simulink model "rakete"  (R2017b)
settings: Solver=ode4  StartTime=0.0  StopTime=600.0  FixedStep=10  RelTol=1e-3
settings Model: Creator=squirrel  LastModifiedBy=squirrel

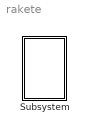
== system rakete ==
  Subsystem : Subsystem  mask{m1_leer=500, m2_leer=1000, St1_Treibstoff=4000, St2_Treibstoff=1500, Durchsatz_1=20, Durchsatz_2=15, SchubProDurchsatz=4000}

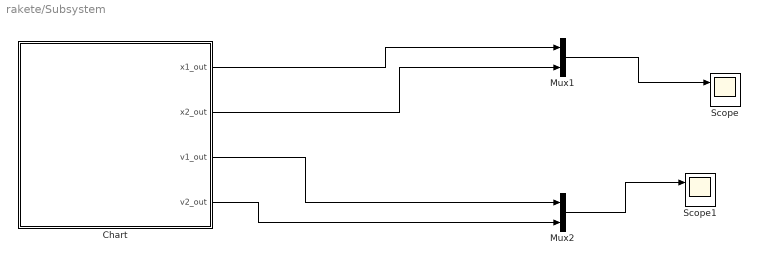
== system rakete/Subsystem ==
  Chart : Stateflow chart  TreatAsAtomicUnit=on
  Mux1 : Mux  Inputs=2
  Mux2 : Mux  Inputs=2
  Scope : Scope  NumInputPorts=2
  Scope1 : Scope  NumInputPorts=2
  wires:
  Mux1/1 -> Scope/1
  Chart/1(x1_out) -> Mux1/1
  Chart/2(x2_out) -> Mux1/2
  Chart/3(v1_out) -> Mux2/1
  Chart/4(v2_out) -> Mux2/2
  Mux2/1 -> Scope1/1

== stateflow chart rakete/Subsystem/Chart ==
  settings: updateMethod=CONTINUOUS
  state StufenGemeinsam
    du:
    %derivatives
    [v1_dot, v2_dot] = acc1();
    x1_dot = v1; x2_dot = v2;
    m1_dot = -Durchsatz_1; m2_dot = 0;
    %output
    x1_out = x1; x2_out = x2;
    v1_out = v1; v2_out = v2;
  state Stufe2Ausgebrannt
    du:
    %derivatives
    [v1_dot, v2_dot] = acc3();
    x1_dot = v1; x2_dot = v2;
    m1_dot = 0; m2_dot = 0;
    %output
    x1_out = x1; x2_out = x2;
    v1_out = v1; v2_out = v2;
  state StufenGetrennt
    du:
    %derivatives
    [v1_dot, v2_dot] = acc2();
    x1_dot = v1; x2_dot = v2;
    m1_dot = 0; m2_dot = -Durchsatz_2;
    %output
    x1_out = x1; x2_out = x2;
    v1_out = v1; v2_out = v2;
  (default) -> StufenGemeinsam : {init();}
  StufenGemeinsam -> StufenGetrennt : [m1 <= m1_leer]
  StufenGetrennt -> Stufe2Ausgebrannt : [m2 <= m2_leer]
  data: a1 function_output; a2 function_output; a1 function_output; a2 function_output; a1 function_output; a2 function_output; m1_leer parameter; m2_leer parameter; St1_Treibstoff parameter; St2_Treibstoff parameter; Durchsatz_1 parameter; Durchsatz_2 parameter; x2 local; v1 local; v2 local; m1 local; m2 local; x1_out output; x2_out output; v1_out output; v2_out output; SchubProDurchsatz parameter double; x1 local; er constant double =6378000; G constant double =66.743 * 10^(-12); me constant double =5.9736 * 10^24
  data x2 settings: updateMethod=SF_CONTINUOUS_TIME_DATA
  data v1 settings: updateMethod=SF_CONTINUOUS_TIME_DATA
  data v2 settings: updateMethod=SF_CONTINUOUS_TIME_DATA
  data m1 settings: updateMethod=SF_CONTINUOUS_TIME_DATA
  data m2 settings: updateMethod=SF_CONTINUOUS_TIME_DATA
  data x1 settings: updateMethod=SF_CONTINUOUS_TIME_DATA
  function init:
    | function init
    | v1 = 0; % Geschwindigkeit Stufe 1 [m/s]
    | v2 = 0; % Geschwindigkeit Stufe 2 [m/s]
    | 
    | m1 = m1_leer + St1_Treibstoff; % initiale Masse Stufe 1 [kg]
    | m2 = m2_leer + St2_Treibstoff; % initiale Masse Stufe 2 [kg]
    | x1 = 0; % Position Stufe 1
    | x2 = 0; % Position Stufe 2
  function [a1, a2] = acc1:
    | function [a1, a2] = acc1
    | 
    | m = m1 + m2 + m1_leer + m2_leer; % aktuelle Gesamtmasse Stufe 1 und 2 [kg]
    | Fg = (G * me * m) / ((er + x1)^2); % Potentialkraft [N]
    | Fs = Durchsatz_1 * SchubProDurchsatz; % Schubkraft [N]
    | 
    | a1 = (Fs - Fg) / m; % Beschleunigung Stufe 1 [m/s^2]
    | a2 = a1; % Beschleunigung Stufe 2 [m/s²]
  function [a1, a2] = acc2:
    | function [a1, a2] = acc2
    | 
    | m = m2 + m2_leer; % aktuelle Gesamtmasse Stufe 2 [kg]
    | 
    | Fg1 = (G * me) / (er + x1)^2; % Potentialkraft Stufe 1[N]
    | 
    | Fg2 = (G * me * m) / (er + x2)^2; % Potentialkraft Stufe 2[N]
    | Fs2 = Durchsatz_2 * SchubProDurchsatz;  % Schubkraft Stufe 2 [N]
    | a1 = - Fg1;  % Beschleunigung Stufe 1 [m/s²]
    | a2 = (Fs2 - Fg2) / m; % Beschleunigung Stufe 2 [m/s²]
  function [a1, a2] = acc3:
    | function [a1, a2] = acc3
    | 
    | Fg1 = (G * me) / (er + x1)^2; % Potentialkraft Stufe 1[N]
    | 
    | Fg2 = (G * me) / (er + x2)^2; % Potentialkraft Stufe 2[N]
    | a1 = - Fg1; % Beschleunigung Stufe 1 [m/s²]
    | a2 = - Fg2; % Beschleunigung Stufe 2 [m/s²]
